simulink library "MSP_MT_lib"  (R2016b)
settings: Solver=VariableStepAuto  StartTime=0.0  StopTime=10.0  RelTol=1e-3
settings Model: Creator=taylorreynolds  LastModifiedBy=Taylor

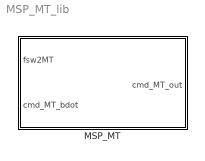
== system MSP_MT_lib ==
  MSP_MT : Subsystem

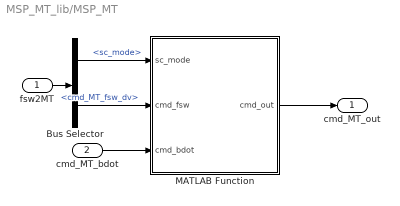
== system MSP_MT_lib/MSP_MT ==
  fsw2MT : Inport  OutDataTypeStr=Bus: fsw2mt
  cmd_MT_bdot : Inport  Port=2
  Bus Selector : BusSelector  OutputSignals=sc_mode,cmd_MT_fsw_dv
  MATLAB Function : MATLAB Function  TreatAsAtomicUnit=on
  cmd_MT_out : Outport
  wires:
  cmd_MT_bdot/1 -> MATLAB Function/3(cmd_bdot)
  MATLAB Function/1(cmd_out) -> cmd_MT_out/1
  fsw2MT/1 -> Bus Selector/1
  Bus Selector/1 -> MATLAB Function/1(sc_mode)  "<sc_mode>"
  Bus Selector/2 -> MATLAB Function/2(cmd_fsw)  "<cmd_MT_fsw_dv>"

== matlab function MSP_MT_lib/MSP_MT/MATLAB Function ==
  data: sc_mode input; cmd_fsw input; cmd_out output int8; cmd_bdot input
function cmd_out = MT_logic(sc_mode,cmd_fsw,cmd_bdot)

% Chooses which control signal to pass through based on the sc_mode
%   mode_logic.bdot             = 1;
%   mode_logic.desat_eclipse    = 2;
%   mode_logic.point            = 3;
%       point.velocity          = 31;
%       point.ground            = 32;
%       point.MPC               = 33;
%   mode_logic.low_power        = 4;

% Note: If sc_mode = 0, then ADCS FSW is assumed to be powered off and the
% bdot command will automatically be passed through

if( sc_mode == 0 ) % ADCS FSW is powered off
    cmd_out = cmd_bdot;
else
    if( sc_mode == 1 ) % ADCS FSW indicates a tumble
        cmd_out = cmd_bdot;
    else
        cmd_out = cmd_fsw; % ADCS FSW wants control
    end
end
